simulink model "vmr_rwd_fix_leftarm"  (R2015a)
settings: Solver=ode4  SolverMode=MultiTasking  StartTime=0.0  StopTime=inf  FixedStep=BKIN_STEP_TIME  RelTol=1e-3
StartFcn:
  |  warndlg('Dexterit-E models cannot run under simulation. Please compile your model and run it from within Dexterit-E.');set_param(bdroot,'SimulationCommand','stop')
model workspace (MAT data in the model file):
  BKIN_STEP_TIME = 0.00025
  col_x = 1
  col_y = 2
  E_TARGET_ON = 3
  LOGICAL_RADIUS = 4
  START_TARGET_COL = 1
  END_TARGET_COL = 2
  ROTATION_CENTER = 3
  MAXREACHTIME_COL = 5
  ROTATION_TYPE = 7
  ROTATION = 8
  DELAY_POSTTRIAL_COL = 6
  E_STAY_CENTER = 2
  VISUAL_RADIUS = 3
  COLOR = 5
  K_SCORETEXT_ROW = 1
  LABEL_HEIGHT = 8
  HITCOLOR = 6
  E_HIT_TARGET = 5
  E_MISS_TARGET = 9
  K_REWARD_VAL = 2
  K_TONE_HIT_DURATION = 4
  K_TONE_HIT_FREQUENCY = 5
  K_VIS_RAD = 6
  E_REWARD = 6
  WAIT_AT_START_COL = 4
  LABEL = 7
  K_RETURN_RING_ROW = 7
  STROKE_WIDTH = 9
  STROKE_COLOR = 10
  K_SCORE_TIME = 8
  HAND_VIS_COL = 9
  CLAMP_COL = 10
  DO_REWARD_COL = 11
  K_TONE_NEUTRAL_DURATION = 10
  K_TONE_NEUTRAL_FREQUENCY = 11
  E_NEUTRAL_FDBK = 10
  E_SHOW_SCORE = 17
  DISPLAY_TRIAL_COL = 12
  K_INSTRUCT_TIME = 9
  E_SHOW_INSTRUCT = 18
  INSTRUCT_PAUSE_BTN = 2
  K_LEFTHAND_TGT = 12
  K_ROBOT_RAMP_TIME = 14
  K_ROBOT_MOVE_TIME = 15
  K_FIX_LEFTHAND = 13
  BKIN_KINEMATIC_FRAME_SIZE = 400
  E_NO_EVENT = 0
  K_UNUSED = 3
  ROTATED_COLOR = 11
undefined symbols (not defined in the file or in its folder): slselsubs
libraries: Video x9, slrtlib x7, General x3, KINARM_general x2, KINARM_loads x2, simulink x1, xpcnilib x1
(part 1 of 2)
CloseFcn:
  | rtwprivate ssgencode ModelCloseRequest b2lab2d
settings Model: ModifiedComment=chris -- Wed Feb 16 09:18:30 2005 -- Version 1.1384  ModifiedHistory=Feb 16/05 - Add error repeat, add offset ramp  ExtModeArmWhenConnect=off  ExtModeLogAll=off  Creator=Chris Grebeldinger  LastModifiedBy=User
settings SolverCC: EnableConcurrentExecution=on  AutoInsertRateTranBlk=on
settings DataIOCC: LimitDataPoints=off  SignalLoggingSaveFormat=ModelDataLogs  SaveOutput=off  SaveTime=off  SignalLoggingName=sigsOut
settings OptimizationCC: BlockReduction=off  BooleanDataType=off  OptimizeBlockIOStorage=off  BufferReuse=off  GlobalBufferReuse=off  ExpressionFolding=off  ExpressionDepthLimit=2147483647  LocalBlockOutputs=off  InitFltsAndDblsToZero=on
settings DebuggingCC: SaveWithParameterizedLinksMsg=none  UnderspecifiedInitializationDetection=Classic  MergeDetectMultiDrivingBlocksExec=none  SignalResolutionControl=TryResolveAllWithWarning  MultiTaskDSMMsg=warning  FcnCallInpInsideContextMsg=UseLocalSettings  StateNameClashWarn=warning  StrictBusMsg=ErrorOnBusTreatedAsVector
settings HardwareCC: ProdIntDivRoundTo=Zero  ProdEndianess=LittleEndian  ProdLongLongMode=on  ProdHWDeviceType=Generic->32-bit x86 compatible  TargetHWDeviceType=32-bit Generic
settings SFSimCC: SimParseCustomCode=off
settings RTWCC: SystemTargetFile=slrt.tlc  TemplateMakefile=slrt_default_tmf  Description=Simulink Real-Time  CustomSourceCode="#include \"stdio.h\""  RTWCompilerOptimization=on
settings CodeAppCC: MaxIdLength=63
settings SimulinkRealTimeCC: TargetFcnLib=ansi_tfl_tmw.mat  GeneratePreprocessorConditionals=Disable all  xPCisDownloadable=off

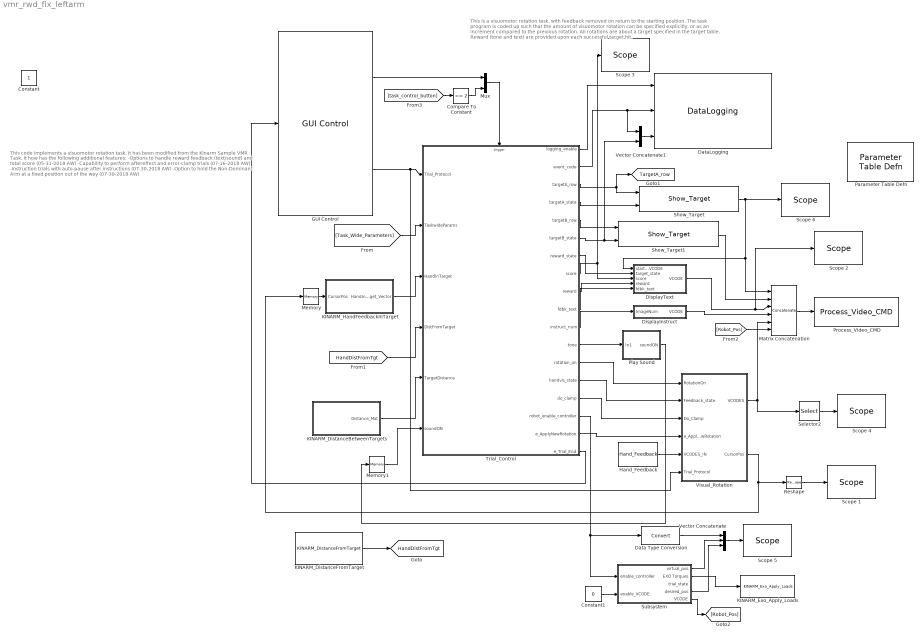
== system vmr_rwd_fix_leftarm ==
  note: This code implements a visuomotor rotation task. It has been modified from the Kinarm Sample VMR Task. It how has the following additional features:
      |
      | -Options to handle reward feedback (text/sound) and total score (05-31-2018 AW)
      | -Capability to perform aftereffect and error-clamp trials (07-16-2018 AW)
      | -Instruction trials with auto-pause after instructions (07-30-2018 AW)
      | -Option to hold the Non-Dominant Arm at a fixed position out of the way (07-30-2018 AW)
  note: This is a visuomotor rotation task, with feedback removed on return to the starting position.
      | The task program is coded up such that the amount of visuomotor rotation can be specified explicitly, or as an increment compared to the previous rotation.
      | All rotations are about a target specified in the target table.
      |
      | Reward (tone and text) are provided upon each successful target hit.
  Compare To Constant : simulink/Logic and Bit Operations/Compare To Constant  relop===  const=2  OutDataTypeStr=boolean
  Constant1 : Constant  Value=0  OutDataTypeStr=boolean
  Data Type Conversion : DataTypeConversion
  DataLogging : General/DataLogging  log_event_codes=on  log_analog_inputs=on  show_time_remaining=off
  DisplayInstruct : Subsystem
  DisplayText : Subsystem
  GUI Control : General/GUI Control  target_type_str=Circle  Target_Type=1  XYcols=[1 2]  Vcols=3  Lcols=4  indices_padding=[0 0 0 0;0 0 0 0]  task_version=1.0  show_repeat_trial_flag=off  target_table_rows=32  load_table_rows=20  tp_table_rows=100
  Hand_Feedback : KINARM_general/Hand_Feedback  feedback_cntl_src=none
  KINARM_DistanceBetweenTargets : Subsystem
  KINARM_DistanceFromTarget : KINARM_general/KINARM_DistanceFromTarget  use_dominant_hand=on
  KINARM_Exo_Apply_Loads : KINARM_loads/KINARM_Exo_Apply_Loads  up_duration=1500  down_duration=1500  max_torque=8  limit_motors=off
  KINARM_HandFeedbackInTarget : Subsystem  AncestorBlock=KINARM_general/KINARM_HandInTarget  mask(KINARM_HandInTarget){use_dominant_hand=on, target_type=Circle, num_states=1, attribcol1=4, attribcol2=3, attribcol3=3, attribcol4=3}
      mask prompts: use_dominant_hand "Dominant Hand?"; target_type "Type of Target"; num_states "Number of Target States"; attribcol1 "State 1 Target Table Column(s)"; attribcol2 "State 2 Target Table Column(s)"; attribcol3 "State 3 Target Table Column(s)"; attribcol4 "State 4 Target Table Column(s)"
      mask help: This block returns a vector or array corresponding to the Target_Table rows indicating whether the specified hand is in (=1) or out (=0) of each of the targets.
      mask init:
      | num_states=str2num(get_param(gcb, 'num_states'));
      | columntext='(columns: ';
      | 
      | for i=1:num_states
      | 	varname=['attribcol' num2str(i)];
      | 	if i>1
      | 		columntext=[columntext, '; '];
      | 	end
      | 	columntext=[columntext, get_param(gcb, varname)];
      | end
      | columntext=strvcat([columntext ')'],' ', ' ');
      | 
      | output_block=char(find_system(gcb,'LookUnderMasks','all','FollowLinks','on','SearchDepth',1,'BlockType','Outport'));
      | outputname=get_param(output_block,'Name');
      | 
      | % Select only the desired states for output. The output port is also renamed to reflect 
      | % whether the output is a vector (in the case of a single state) or an array (of vectors, 
      | % one for each of multiple states).
      | if num_states == 1
      | 	set_param([gcb '/Selected States'], 'Value', '[1]');
      | 	set_param(output_block, 'Name', 'HandInTarget_Vector');
      | elseif num_states == 2
      | 	set_param([gcb '/Selected States'], 'Value', '[1,2]');
      | 	set_param(output_block, 'Name', 'HandInTarget_Array');
      | elseif num_states == 3
      | 	set_param([gcb '/Selected States'], 'Value', '[1,2,3]');
      | 	set_param(output_block, 'Name', 'HandInTarget_Array');
      | else
      | 	set_param([gcb '/Selected States'], 'Value', '[1,2,3,4]');
      | 	set_param(output_block, 'Name', 'HandInTarget_Array');
      | end
      mask Help:
      | Used to determine if the hand (finger-tip) is in any of the targets in the Target_Table.
      | <P>
      | <B><I>Use of this block requires that the DataLogging block (General library) be set to log KINARM data.</I></B>
      | 
      | <H2>Library </H2>
      | KINARM_general (sub-library)
      | 
      | <H2>Description </H2>
      | This block returns a vector or array corresponding to the Target_Table rows indicating whether the specified hand (i.e. finger-tip) is in or out of each of the targets.  Each element in the output vector or output array will be either a 0 (hand not in target) or a 1 (hand in target).
      | <P>
      | A vector is returned if only one target state is specified in each target row (see Parameters and Dialog Box), with each index of the vector corresponding to a row in the target table.  An array is returned if more than one target state is specified in a target row, with each row of the array corresponding to a target row and each column corresponding to the nth target state specified in each target row.
      | <P>
      | The output vector or array is typically used by a stateflow chart to affect behavior of the system.  Because this block returns hand-in-target information for all targets in the target table, multiple targets can be monitored at once (i.e. the stateflow chart could have certain transitions that occur if the hand is in one target and other transitions if it is in a different target).  Likewise, because this block returns hand-in-target information for multiple states of a single target, those multiple states can be monitored simultaneously.
      | <P>
      | Because the KINARM_HandInTarget block returns information for only one hand, two copies of this block are required if information for both hands is desired.
      | <P>
      | 
      | <H2>Parameters and Dialog Box</H2>
      | <B>Dominant Hand?:</B> this box determines which hand is used by this block : dominant hand position (checked box) or the non-dominant hand position (unchecked box).  (Note: if the end-user wants to know about both the dominant hand and the non-dominant hand, then 2 separate copies of this block are requried, one for each hand.)
      | <P>
      | <B>Type of Target:</B> Enter the type of target specified in the target table:
      | <P>
      | <B>Number of Target States:</B> Enter the number of target states specified in each target row.  Up to four target states are allowed per target row.
      | <P>
      | <B>State <n> Target Table Columns:</B> Enter the columns in the Target Table that specify the relevant target attributes.  Do this for each target state.
      | For a circle, enter the columns corresponding to logical radius (e.g. 4)
      | <BR>For an ellipse, enter the columns corresponding to major radius, minor radius, rotation angle (e.g. [4, 5, 6]).
      | <BR>For a rectangle, enter the columns corresponding to length, height, and rotation angle (e.g. [4, 5, 6]).
      | <BR>For a line, enter the columns corresponding to stroke width, endpoint in x, and endpoint in y (e.g. [3, 4, 5]).
      | <BR>For a triangle, enter the columns corresponding to length, height, peak offset, and rotation angle (e.g. [4, 5, 6, 7]).
      | 
      | <H2>Examples</H2>
      | <B>Example 1.</B>  Suppose a target row will be used to define 1 state for a circle type target and the radius of the visual target is the same radius to be used for determination of hand-in-target.  The related Target Table column is: column 6 = radius.  For this example, "State 1 Target Table Columns" would equal [6].
      | <P>
      | 
      | <B>Example 2.</B>  Suppose a target row will be used to define 1 state for a circle type target, but the radius of the visual target will be different than the radius to be used for determination of hand-in-target.  This option allows independent control over the size of the visual target versus the accuracy needed to be considered "in the target".  The related Target Table columns are: column 6 = radius1 (i.e. radius to target to be drawn); column 7 = radius2 (i.e. radius to be used for hand-in-target) .  For this example, "State 1 Target Table Columns" would equal [7].
      | <P>
      | <B>Example 3.</B>  Suppose a target row will be used to define 2 states for a circle type target, where the radius of the visual target will be a constant, but depending on the state of the system, one of 2 other and different radii will be used for determination of hand-in-target.  The related Target Table columns are: column 6 = radius1 (i.e. radius to target to be drawn); column 7 = radius2 (i.e. radius to be used for hand-in-target for state 1); column 8 = radius3 (i.e. radius to be used for hand-in-target for state 2).  For this example, "State 1 Target Table Columns" would equal [7], while "State 2 Target Table Columns" would equal [8].
      | <P>
      | 
      | <H2>Related Blocks </H2>
      | DataLogging
      mask TypeOptions target_type: Circle | Ellipse | Rectangle | Line | Triangle
      mask Callback target_type:
      | target_type=get_param(gcb, 'target_type');
      | attribcol1=[str2num(get_param(gcb, 'attribcol1')) 0 0 0 0 0 0];
      | attribcol2=[str2num(get_param(gcb, 'attribcol2')) 0 0 0 0 0 0];
      | attribcol3=[str2num(get_param(gcb, 'attribcol3')) 0 0 0 0 0 0];
      | attribcol4=[str2num(get_param(gcb, 'attribcol4')) 0 0 0 0 0 0];
      | switch target_type(1:3)
      | 	case 'Cir'
      | 		numcol=1;
      | 	case 'Ell'
      | 		numcol=3;
      |     case 'Rec'
      |         numcol=3;
      |     case 'Lin'
      |         numcol=3;
      |     case 'Tri'
      |         numcol=4;
      | 	otherwise
      | 		numcol=1;
      | end
      | if numcol==1
      | 	set_param(gcb, 'attribcol1', num2str(attribcol1(1)));
      | 	set_param(gcb, 'attribcol2', num2str(attribcol2(1)));
      | 	set_param(gcb, 'attribcol3', num2str(attribcol3(1)));
      | 	set_param(gcb, 'attribcol4', num2str(attribcol4(1)));
      | else
      | 	set_param(gcb, 'attribcol1', ['[' num2str(attribcol1(1:numcol)) ']']);
      | 	set_param(gcb, 'attribcol2', ['[' num2str(attribcol2(1:numcol)) ']']);
      | 	set_param(gcb, 'attribcol3', ['[' num2str(attribcol3(1:numcol)) ']']);
      | 	set_param(gcb, 'attribcol4', ['[' num2str(attribcol4(1:numcol)) ']']);
      | end
      mask TypeOptions num_states: 1 | 2 | 3 | 4
      mask Callback num_states:
      | num_states = str2num(get_param(gcb, 'num_states'));
      | vis = get_param(gcb, 'MaskVisibilities');
      | 
      | % Select only the desired states for output. The output port is also renamed to reflect
      | % whether the output is a vector (in the case of a single state) or an array (of vectors,
      | % one for each of multiple states).
      | output_block=char(find_system(gcb, 'LookUnderMasks', 'all', 'FollowLinks', 'on', 'SearchDepth', 1, 'BlockType', 'Outport'));
      | 
      | if num_states == 1
      | 	set_param([gcb '/Selected States'], 'Value', '[1]');
      | 	set_param(output_block, 'Name', 'HandInTarget_Vector');
      | 	vis{5} = 'off';
      | 	vis{6} = 'off';
      | 	vis{7} = 'off';
      | elseif num_states == 2
      | 	set_param([gcb '/Selected States'], 'Value', '[1,2]');
      | 	set_param(output_block, 'Name', 'HandInTarget_Array');
      | 	vis{5} = 'on';
      | 	vis{6} = 'off';
      | 	vis{7} = 'off';
      | elseif num_states == 3
      | 	set_param([gcb '/Selected States'], 'Value', '[1,2,3]');
      | 	set_param(output_block, 'Name','HandInTarget_Array');
      | 	vis{5} = 'on';
      | 	vis{6} = 'on';
      | 	vis{7} = 'off';
      | else
      | 	set_param([gcb '/Selected States'], 'Value', '[1,2,3,4]');
      | 	set_param(output_block, 'Name', 'HandInTarget_Array');
      | 	vis{5} = 'on';
      | 	vis{6} = 'on';
      | 	vis{7} = 'on';
      | end
      | set_param(gcb, 'MaskVisibilities', vis);
      | 
      | target_type=get_param(gcb, 'target_type');
      | attribcol1=[str2num(get_param(gcb, 'attribcol1')) 0 0 0 0 0 0];
      | attribcol2=[str2num(get_param(gcb, 'attribcol2')) 0 0 0 0 0 0];
      | attribcol3=[str2num(get_param(gcb, 'attribcol3')) 0 0 0 0 0 0];
      | attribcol4=[str2num(get_param(gcb, 'attribcol4')) 0 0 0 0 0 0];
      | switch target_type(1:3)
      | 	case 'Cir'
      | 		numcol=1;
      | 	case 'Ell'
      | 		numcol=3;
      |     case 'Rec'
      |         numcol=3;
      |     case 'Lin'
      |         numcol=3;
      |     case 'Tri'
      |         numcol=4;
      | 	otherwise
      | 		numcol=1;
      | end
      | if numcol==1
      | 	set_param(gcb, 'attribcol1', num2str(attribcol1(1)));
      | 	set_param(gcb, 'attribcol2', num2str(attribcol2(1)));
      | 	set_param(gcb, 'attribcol3', num2str(attribcol3(1)));
      | 	set_param(gcb, 'attribcol4', num2str(attribcol4(1)));
      | else
      | 	set_param(gcb, 'attribcol1', ['[' num2str(attribcol1(1:numcol)) ']']);
      | 	set_param(gcb, 'attribcol2', ['[' num2str(attribcol2(1:numcol)) ']']);
      | 	set_param(gcb, 'attribcol3', ['[' num2str(attribcol3(1:numcol)) ']']);
      | 	set_param(gcb, 'attribcol4', ['[' num2str(attribcol4(1:numcol)) ']']);
      | end
      mask Callback attribcol1:
      | target_type=get_param(gcb, 'target_type');
      | attribcol1=[str2num(get_param(gcb, 'attribcol1')) 0 0 0 0 0 0];
      | attribcol2=[str2num(get_param(gcb, 'attribcol2')) 0 0 0 0 0 0];
      | attribcol3=[str2num(get_param(gcb, 'attribcol3')) 0 0 0 0 0 0];
      | attribcol4=[str2num(get_param(gcb, 'attribcol4')) 0 0 0 0 0 0];
      | switch target_type(1:3)
      | 	case 'Cir'
      | 		numcol=1;
      | 	case 'Ell'
      | 		numcol=3;
      |     case 'Rec'
      |         numcol=3;
      |     case 'Lin'
      |         numcol=3;
      |     case 'Tri'
      |         numcol=4;
      | 	otherwise
      | 		numcol=1;
      | end
      | if numcol==1
      | 	set_param(gcb, 'attribcol1', num2str(attribcol1(1)));
      | 	set_param(gcb, 'attribcol2', num2str(attribcol2(1)));
      | 	set_param(gcb, 'attribcol3', num2str(attribcol3(1)));
      | 	set_param(gcb, 'attribcol4', num2str(attribcol4(1)));
      | else
      | 	set_param(gcb, 'attribcol1', ['[' num2str(attribcol1(1:numcol)) ']']);
      | 	set_param(gcb, 'attribcol2', ['[' num2str(attribcol2(1:numcol)) ']']);
      | 	set_param(gcb, 'attribcol3', ['[' num2str(attribcol3(1:numcol)) ']']);
      | 	set_param(gcb, 'attribcol4', ['[' num2str(attribcol4(1:numcol)) ']']);
      | end
      mask Callback attribcol2:
      | target_type=get_param(gcb, 'target_type');
      | attribcol1=[str2num(get_param(gcb, 'attribcol1')) 0 0 0 0 0 0];
      | attribcol2=[str2num(get_param(gcb, 'attribcol2')) 0 0 0 0 0 0];
      | attribcol3=[str2num(get_param(gcb, 'attribcol3')) 0 0 0 0 0 0];
      | attribcol4=[str2num(get_param(gcb, 'attribcol4')) 0 0 0 0 0 0];
      | switch target_type(1:3)
      | 	case 'Cir'
      | 		numcol=1;
      | 	case 'Ell'
      | 		numcol=3;
      |     case 'Rec'
      |         numcol=3;
      |     case 'Lin'
      |         numcol=3;
      |     case 'Tri'
      |         numcol=4;
      | 	otherwise
      | 		numcol=1;
      | end
      | if numcol==1
      | 	set_param(gcb, 'attribcol1', num2str(attribcol1(1)));
      | 	set_param(gcb, 'attribcol2', num2str(attribcol2(1)));
      | 	set_param(gcb, 'attribcol3', num2str(attribcol3(1)));
      | 	set_param(gcb, 'attribcol4', num2str(attribcol4(1)));
      | else
      | 	set_param(gcb, 'attribcol1', ['[' num2str(attribcol1(1:numcol)) ']']);
      | 	set_param(gcb, 'attribcol2', ['[' num2str(attribcol2(1:numcol)) ']']);
      | 	set_param(gcb, 'attribcol3', ['[' num2str(attribcol3(1:numcol)) ']']);
      | 	set_param(gcb, 'attribcol4', ['[' num2str(attribcol4(1:numcol)) ']']);
      | end
      mask Callback attribcol3:
      | target_type=get_param(gcb, 'target_type');
      | attribcol1=[str2num(get_param(gcb, 'attribcol1')) 0 0 0 0 0 0];
      | attribcol2=[str2num(get_param(gcb, 'attribcol2')) 0 0 0 0 0 0];
      | attribcol3=[str2num(get_param(gcb, 'attribcol3')) 0 0 0 0 0 0];
      | attribcol4=[str2num(get_param(gcb, 'attribcol4')) 0 0 0 0 0 0];
      | switch target_type(1:3)
      | 	case 'Cir'
      | 		numcol=1;
      | 	case 'Ell'
      | 		numcol=3;
      |     case 'Rec'
      |         numcol=3;
      |     case 'Lin'
      |         numcol=3;
      |     case 'Tri'
      |         numcol=4;
      | 	otherwise
      | 		numcol=1;
      | end
      | if numcol==1
      | 	set_param(gcb, 'attribcol1', num2str(attribcol1(1)));
      | 	set_param(gcb, 'attribcol2', num2str(attribcol2(1)));
      | 	set_param(gcb, 'attribcol3', num2str(attribcol3(1)));
      | 	set_param(gcb, 'attribcol4', num2str(attribcol4(1)));
      | else
      | 	set_param(gcb, 'attribcol1', ['[' num2str(attribcol1(1:numcol)) ']']);
      | 	set_param(gcb, 'attribcol2', ['[' num2str(attribcol2(1:numcol)) ']']);
      | 	set_param(gcb, 'attribcol3', ['[' num2str(attribcol3(1:numcol)) ']']);
      | 	set_param(gcb, 'attribcol4', ['[' num2str(attribcol4(1:numcol)) ']']);
      | end
      mask Callback attribcol4:
      | target_type=get_param(gcb, 'target_type');
      | attribcol1=[str2num(get_param(gcb, 'attribcol1')) 0 0 0 0 0 0];
      | attribcol2=[str2num(get_param(gcb, 'attribcol2')) 0 0 0 0 0 0];
      | attribcol3=[str2num(get_param(gcb, 'attribcol3')) 0 0 0 0 0 0];
      | attribcol4=[str2num(get_param(gcb, 'attribcol4')) 0 0 0 0 0 0];
      | switch target_type(1:3)
      | 	case 'Cir'
      | 		numcol=1;
      | 	case 'Ell'
      | 		numcol=3;
      |     case 'Rec'
      |         numcol=3;
      |     case 'Lin'
      |         numcol=3;
      |     case 'Tri'
      |         numcol=4;
      | 	otherwise
      | 		numcol=1;
      | end
      | if numcol==1
      | 	set_param(gcb, 'attribcol1', num2str(attribcol1(1)));
      | 	set_param(gcb, 'attribcol2', num2str(attribcol2(1)));
      | 	set_param(gcb, 'attribcol3', num2str(attribcol3(1)));
      | 	set_param(gcb, 'attribcol4', num2str(attribcol4(1)));
      | else
      | 	set_param(gcb, 'attribcol1', ['[' num2str(attribcol1(1:numcol)) ']']);
      | 	set_param(gcb, 'attribcol2', ['[' num2str(attribcol2(1:numcol)) ']']);
      | 	set_param(gcb, 'attribcol3', ['[' num2str(attribcol3(1:numcol)) ']']);
      | 	set_param(gcb, 'attribcol4', ['[' num2str(attribcol4(1:numcol)) ']']);
      | end
      mask Display:
      | disp(columntext)
      | port_label('output',1,outputname)
  Matrix Concatenation : Concatenate  NumInputs=6  Mode=Multidimensional array
  Memory : Memory  InheritSampleTime=on
  Memory1 : Memory  LinearizeMemory=on
  Mux : Mux  Inputs=2
  Parameter Table Defn : General/Parameter Table Defn  ShowInLibBrowser=0
  Play Sound : Subsystem
  Process_Video_CMD : Video/Process_Video_CMD  video_delay=50
  Reshape : Reshape
  Scope 1 : slrtlib/Displays and Logging/Scope   scopeno=6  scopetype=Target  autostart=on  viewmode=Numerical  formatstr='%15.6f'  grid=on  ylimits=[0,0]  nosamples=250  noprepostsamples=0  interleave=1  triggermode=FreeRun  triggersignal=1  trigsignalfromport=off  triggerlevel=0.0  triggerslope=Either  triggerscope=1  triggersample=0  filename=data.dat  mode=Lazy  writesize=512  autorestart=off  dynamicfilemode=off  maxwritefilesize=512*1024^2
  Scope 2 : slrtlib/Displays and Logging/Scope   scopeno=1  scopetype=Target  autostart=on  viewmode=Numerical  formatstr='%15.6f'  grid=on  ylimits=[0,0]  nosamples=250  noprepostsamples=0  interleave=1  triggermode=FreeRun  triggersignal=1  trigsignalfromport=off  triggerlevel=0.0  triggerslope=Either  triggerscope=1  triggersample=0  filename=data.dat  mode=Lazy  writesize=512  autorestart=off  dynamicfilemode=off  maxwritefilesize=512*1024^2
  Scope 3 : slrtlib/Displays and Logging/Scope   scopeno=3  scopetype=Target  autostart=on  viewmode=Numerical  formatstr='%15.6f'  grid=on  ylimits=[0,0]  nosamples=250  noprepostsamples=0  interleave=1  triggermode=FreeRun  triggersignal=1  trigsignalfromport=off  triggerlevel=0.0  triggerslope=Either  triggerscope=1  triggersample=0  filename=data.dat  mode=Lazy  writesize=512  autorestart=off  dynamicfilemode=off  maxwritefilesize=512*1024^2
  Scope 4 : slrtlib/Displays and Logging/Scope   scopeno=5  scopetype=Target  autostart=on  viewmode=Numerical  formatstr='%15.6f'  grid=on  ylimits=[0,0]  nosamples=250  noprepostsamples=0  interleave=1  triggermode=FreeRun  triggersignal=1  trigsignalfromport=off  triggerlevel=0.0  triggerslope=Either  triggerscope=1  triggersample=0  filename=data.dat  mode=Lazy  writesize=512  autorestart=off  dynamicfilemode=off  maxwritefilesize=512*1024^2
  Scope 5 : slrtlib/Displays and Logging/Scope   scopeno=2  scopetype=Target  autostart=on  viewmode=Numerical  formatstr='%15.6f'  grid=on  ylimits=[0,0]  nosamples=250  noprepostsamples=0  interleave=1  triggermode=FreeRun  triggersignal=1  trigsignalfromport=off  triggerlevel=0.0  triggerslope=Either  triggerscope=1  triggersample=0  filename=data.dat  mode=Lazy  writesize=512  autorestart=off  dynamicfilemode=off  maxwritefilesize=512*1024^2
  Scope 6 : slrtlib/Displays and Logging/Scope   scopeno=4  scopetype=Target  autostart=on  viewmode=Numerical  formatstr='%15.6f'  grid=on  ylimits=[0,0]  nosamples=250  noprepostsamples=0  interleave=1  triggermode=FreeRun  triggersignal=1  trigsignalfromport=off  triggerlevel=0.0  triggerslope=Either  triggerscope=1  triggersample=0  filename=data.dat  mode=Lazy  writesize=512  autorestart=off  dynamicfilemode=off  maxwritefilesize=512*1024^2
  Selector2 : Selector  NumberOfDimensions=2  InputPortWidth=70  IndexOptions=Index vector (dialog),Select all  Indices=1,1  OutputSizes=1,1
  Show_Target : Video/Show_Target  target_type=Circle  num_states=2  attribcol1=[COLOR 0 0 VISUAL_RADIUS]  attribcol2=[HITCOLOR 0 0 VISUAL_RADIUS]  attribcol3=[0 0 0 0]  attribcol4=[0 0 0 0]  attribcol5=[0 0 24 0]  stateindices_padding=[0 0 0 0 0 0 0;0 0 0 0 0 0 0;0 0 0 0 0 0 0;0 0 0 0 0 0 0;0 0 0 0 0 0 0]  source=dialog  opacity=100  target_display=Both subject and operator displays  num_col=4
  Show_Target1 : Video/Show_Target  target_type=Circle  num_states=3  attribcol1=[COLOR 0 0 VISUAL_RADIUS]  attribcol2=[HITCOLOR 0 0 VISUAL_RADIUS]  attribcol3=[ROTATED_COLOR 0 0 VISUAL_RADIUS]  attribcol4=[0 0 0 0]  attribcol5=[0 0 24 0]  stateindices_padding=[0 0 0 0 0 0 0;0 0 0 0 0 0 0;0 0 0 0 0 0 0;0 0 0 0 0 0 0;0 0 0 0 0 0 0]  source=dialog  opacity=100  target_display=Both subject and operator displays  num_col=4
  Subsystem : Subsystem
  Trial_Control : Stateflow chart  TreatAsAtomicUnit=on
  Vector Concatenate : Concatenate  NumInputs=3
  Vector Concatenate1 : Concatenate
  Visual_Rotation : Subsystem
  Constant : Constant  IOType=siggen
  tag scope: HandDistFromTgt=global, TargetA_row=global
  wires:
  Show_Target/1 -> Scope 6/1, Matrix Concatenation/1, DisplayText/1(start_tgt_VCODE)
  GUI Control/2 -> Visual_Rotation/6(Trial_Protocol), Trial_Control/1(Trial_Protocol)
  Trial_Control/18(e_Trial_End) -> GUI Control/1
  Trial_Control/4(targetA_state) -> Show_Target/2
  Trial_Control/3(targetA_row) -> Show_Target/1, [TargetA_row]
  Show_Target1/1 -> Matrix Concatenation/2
  Trial_Control/5(targetB_row) -> Show_Target1/1
  Trial_Control/6(targetB_state) -> Vector Concatenate1/2, Show_Target1/2
  Trial_Control/2(event_code) -> DataLogging/2, Vector Concatenate1/1
  Matrix Concatenation/1 -> Process_Video_CMD/1
  Hand_Feedback/1 -> Visual_Rotation/5(VCODES_IN)
  Visual_Rotation/2(CursorPos) -> Memory/1, Reshape/1
  KINARM_HandFeedbackInTarget/1(HandInTarget_Vector) -> Trial_Control/3(HandInTarget)
  Trial_Control/17(e_ApplyNewRotation) -> Visual_Rotation/4(e_ApplyNewRotation)
  Trial_Control/1(logging_enable) -> DataLogging/1
  Trial_Control/7(reward_state) -> DisplayText/2(target_state)
  Trial_Control/8(score) -> DisplayText/3(score), Scope 3/1
  [Task_Wide_Parameters] -> Trial_Control/2(TaskwideParams)
  [HandDistFromTgt] -> Trial_Control/4(DistFromTarget)
  KINARM_DistanceBetweenTargets/1(Distance_Mat) -> Trial_Control/5(TargetDistance)
  Trial_Control/9(reward) -> DisplayText/4(reward)
  Trial_Control/13(rotation_on) -> Visual_Rotation/1(RotationOn)
  Trial_Control/14(handvis_state) -> Visual_Rotation/2(Feedback_state)
  Reshape/1 -> Scope 1/1
  Memory/1 -> KINARM_HandFeedbackInTarget/1(CursorPos)
  Selector2/1 -> Scope 4/1
  KINARM_DistanceFromTarget/1 -> [HandDistFromTgt]
  Trial_Control/15(do_clamp) -> Visual_Rotation/3(Do_Clamp)
  DisplayInstruct/1(VCODE) -> Matrix Concatenation/4
  Trial_Control/11(instruct_num) -> DisplayInstruct/1(ImageNum)
  Trial_Control/10(fdbk_text) -> DisplayText/5(fdbk_text)
  Visual_Rotation/1(VCODES) -> Matrix Concatenation/5, Selector2/1
  DisplayText/1(VCODE) -> Scope 2/1, Matrix Concatenation/3
  GUI Control/1 -> Mux/1
  [task_control_button] -> Compare To Constant/1
  Compare To Constant/1 -> Mux/2
  Mux/1 -> Trial_Control/Trigger
  Subsystem/2(EXO Torques) -> KINARM_Exo_Apply_Loads/1
  Subsystem/1(virtual_pos) -> Vector Concatenate/2
  Trial_Control/16(robot_enable_controller) -> Data Type Conversion/1, Subsystem/1(enable_controller)
  Vector Concatenate/1 -> Scope 5/1
  Data Type Conversion/1 -> Vector Concatenate/1
  Subsystem/4(desired_pos) -> Vector Concatenate/3
  Constant1/1 -> Subsystem/2(enable_VCODE)
  Subsystem/5(VCODE) -> [Robot_Pos]
  [Robot_Pos] -> Matrix Concatenation/6
  Vector Concatenate1/1 -> DataLogging/3
  Trial_Control/12(tone) -> Play Sound/1(In1)
  Play Sound/1(soundON) -> Memory1/1
  Memory1/1 -> Trial_Control/6(soundON)

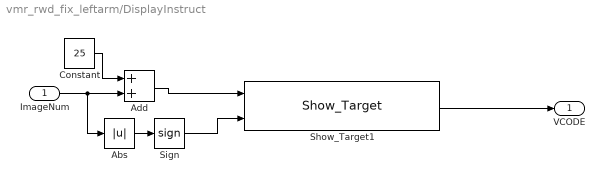
== system vmr_rwd_fix_leftarm/DisplayInstruct ==
  ImageNum : Inport
  Abs : Abs
  Add : Sum
  Constant : Constant  Value=25
  Show_Target1 : Video/Show_Target  target_type=Rectangle  num_states=1  attribcol1=[COLOR 0 0 VISUAL_RADIUS LABEL_HEIGHT 0]  attribcol2=[HITCOLOR 0 0 VISUAL_RADIUS 0 0]  attribcol3=[0 0 0 0 0 0]  attribcol4=[0 0 0 0 0 0]  attribcol5=[0 0 24 0 0 0]  stateindices_padding=[0 0 0 0 0;0 0 0 0 0;0 0 0 0 0;0 0 0 0 0;0 0 0 0 0]  source=dialog  opacity=100  target_display=Both subject and operator displays  num_col=6
  Sign : Signum
  VCODE : Outport
  wires:
  ImageNum/1 -> Add/2, Abs/1
  Abs/1 -> Sign/1
  Sign/1 -> Show_Target1/2
  Show_Target1/1 -> VCODE/1
  Add/1 -> Show_Target1/1
  Constant/1 -> Add/1

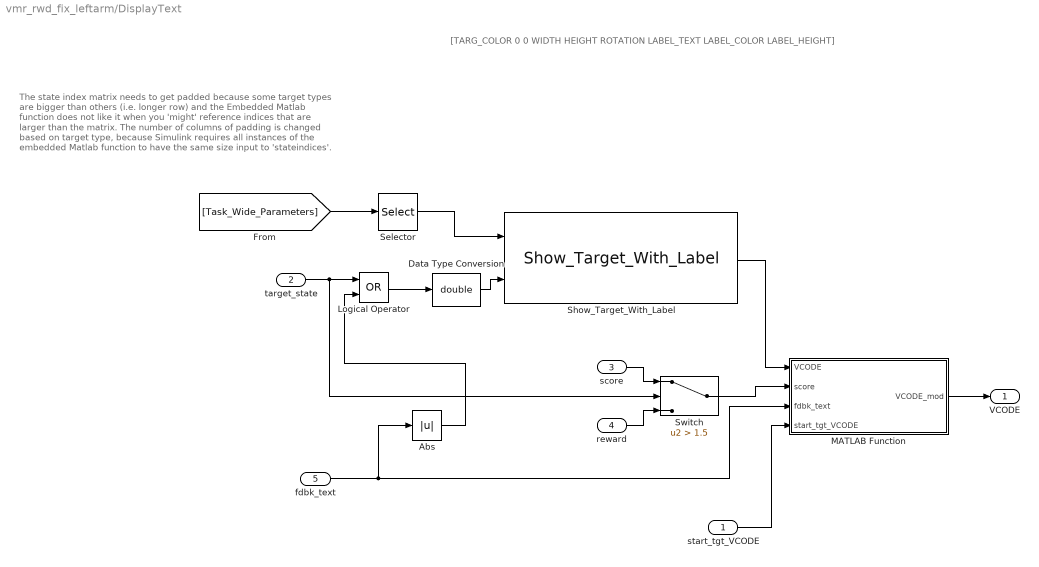
== system vmr_rwd_fix_leftarm/DisplayText ==
  note: [TARG_COLOR 0 0 WIDTH HEIGHT ROTATION LABEL_TEXT LABEL_COLOR LABEL_HEIGHT]
  note: The state index matrix needs to get padded because
      | some target types are bigger than others (i.e. longer row)
      | and the Embedded Matlab function does not like it when you
      |  'might' reference indices that are larger than the matrix.
      |
      | The number of columns of padding is changed based on target
      | type, because Simulink requires all instances of the embedded
      | Matlab function to have the same size input to 'stateindices'.
  start_tgt_VCODE : Inport  OutDataTypeStr=double
  target_state : Inport  Port=2  OutDataTypeStr=double
  score : Inport  Port=3  OutDataTypeStr=int32
  reward : Inport  Port=4  OutDataTypeStr=int32
  fdbk_text : Inport  Port=5  OutDataTypeStr=int32
  Abs : Abs
  Data Type Conversion : DataTypeConversion  OutDataTypeStr=double
  Logical Operator : Logic  Operator=OR  AllPortsSameDT=off  OutDataTypeStr=boolean
  MATLAB Function : MATLAB Function  TreatAsAtomicUnit=on
  Selector : Selector  Indices=[K_SCORETEXT_ROW]
  Show_Target_With_Label : Video/Show_Target_With_Label  target_type=Rectangle  num_states=1  attribcol1=[COLOR 0 0 VISUAL_RADIUS VISUAL_RADIUS 0 LABEL COLOR LABEL_HEIGHT]  attribcol2=[COLOR 0 0 VISUAL_RADIUS VISUAL_RADIUS 0 LABEL COLOR LABEL_HEIGHT]  attribcol3=[0 0 0 0 0 0 0 0 0]  attribcol4=[0 0 0 0 0 0 0 0 0]  attribcol5=[0 0 24 0 0 0 0 0 0]  stateindices_padding=[0 0;0 0;0 0;0 0;0 0]  source=dialog  opacity=100  target_display=Both subject and operator displays
  Switch : Switch  Criteria=u2 > Threshold  Threshold=1.5
  VCODE : Outport
  wires:
  target_state/1 -> Logical Operator/1, Switch/2
  Show_Target_With_Label/1 -> MATLAB Function/1(VCODE)
  MATLAB Function/1(VCODE_mod) -> VCODE/1
  score/1 -> Switch/1
  reward/1 -> Switch/3
  Switch/1 -> MATLAB Function/2(score)
  [Task_Wide_Parameters] -> Selector/1
  Selector/1 -> Show_Target_With_Label/1
  fdbk_text/1 -> Abs/1, MATLAB Function/3(fdbk_text)
  Abs/1 -> Logical Operator/2
  Logical Operator/1 -> Data Type Conversion/1
  Data Type Conversion/1 -> Show_Target_With_Label/2
  start_tgt_VCODE/1 -> MATLAB Function/4(start_tgt_VCODE)

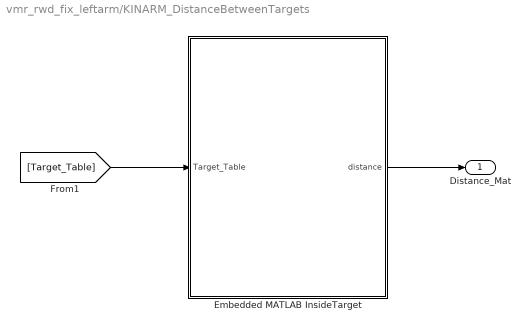
== system vmr_rwd_fix_leftarm/KINARM_DistanceBetweenTargets ==
  Embedded MATLAB InsideTarget : MATLAB Function  TreatAsAtomicUnit=on
  Distance_Mat : Outport
  wires:
  Embedded MATLAB InsideTarget/1(distance) -> Distance_Mat/1
  [Target_Table] -> Embedded MATLAB InsideTarget/1(Target_Table)

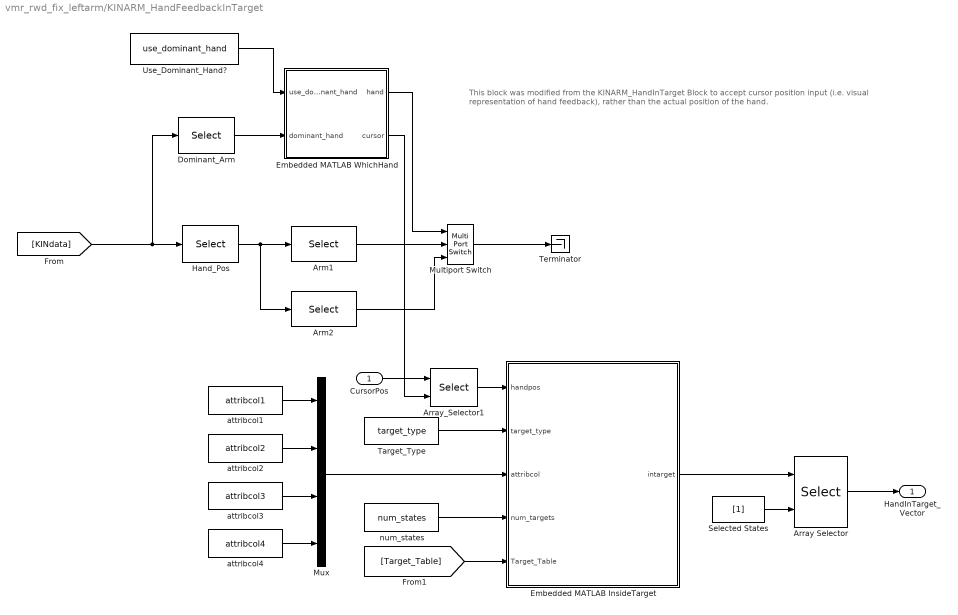
== system vmr_rwd_fix_leftarm/KINARM_HandFeedbackInTarget ==
  note: This block was modified from the KINARM_HandInTarget Block to accept cursor position input (i.e. visual
      | representation of hand feedback), rather than the actual position of the hand.
  CursorPos : Inport
  Arm1 : Selector  NumberOfDimensions=2  InputPortWidth=3  IndexOptions=Index vector (dialog),Select all  Indices=1,-1  OutputSizes=slselsubs([(-2),(-2)],1),slselsubs([(-2),(-2)],2)
  Arm2 : Selector  NumberOfDimensions=2  InputPortWidth=3  IndexOptions=Index vector (dialog),Select all  Indices=2,-1  OutputSizes=slselsubs([(-2),(-2)],1),slselsubs([(-2),(-2)],2)
  Array Selector : Selector  NumberOfDimensions=2  InputPortWidth=3  IndexOptions=Select all,Index vector (port)  Indices=-1,1  OutputSizes=slselsubs([(-2),(-2)],1),slselsubs([(-2),(-2)],2)
  Array_Selector1 : Selector  NumberOfDimensions=2  InputPortWidth=3  IndexOptions=Index vector (port),Select all  Indices=-1,1
  Dominant_Arm : Selector  NumberOfDimensions=2  InputPortWidth=3  IndexOptions=Index vector (dialog),Index vector (dialog)  Indices=[3],[1]  OutputSizes=slselsubs([(-2),(-2)],1),slselsubs([(-2),(-2)],2)
  Embedded MATLAB InsideTarget : MATLAB Function  TreatAsAtomicUnit=on
  Embedded MATLAB WhichHand : MATLAB Function  TreatAsAtomicUnit=on
  Hand_Pos : Selector  NumberOfDimensions=2  InputPortWidth=3  IndexOptions=Select all,Index vector (dialog)  Indices=-1,[23,24]  OutputSizes=slselsubs([(-2),(-2)],1),slselsubs([(-2),(-2)],2)
  Multiport Switch : MultiPortSwitch  Inputs=2
  Mux : Mux
  Selected States : Constant  Value=[1]
  Target_Type : Constant  Value=target_type
  Terminator : Terminator
  Use_Dominant_Hand? : Constant  Value=use_dominant_hand
  attribcol1 : Constant  Value=attribcol1
  attribcol2 : Constant  Value=attribcol2
  attribcol3 : Constant  Value=attribcol3
  attribcol4 : Constant  Value=attribcol4
  num_states : Constant  Value=num_states
  HandInTarget_Vector : Outport
  wires:
  Selected States/1 -> Array Selector/2
  num_states/1 -> Embedded MATLAB InsideTarget/4(num_targets)
  Mux/1 -> Embedded MATLAB InsideTarget/3(attribcol)
  attribcol4/1 -> Mux/4
  attribcol3/1 -> Mux/3
  attribcol2/1 -> Mux/2
  attribcol1/1 -> Mux/1
  Use_Dominant_Hand?/1 -> Embedded MATLAB WhichHand/1(use_dominant_hand)
  Embedded MATLAB WhichHand/1(hand) -> Multiport Switch/1
  Target_Type/1 -> Embedded MATLAB InsideTarget/2(target_type)
  Array Selector/1 -> HandInTarget_Vector/1
  [Target_Table] -> Embedded MATLAB InsideTarget/5(Target_Table)
  Embedded MATLAB InsideTarget/1(intarget) -> Array Selector/1
  Multiport Switch/1 -> Terminator/1
  Arm2/1 -> Multiport Switch/3
  Arm1/1 -> Multiport Switch/2
  Dominant_Arm/1 -> Embedded MATLAB WhichHand/2(dominant_hand)
  Hand_Pos/1 -> Arm2/1, Arm1/1
  [KINdata] -> Dominant_Arm/1, Hand_Pos/1
  CursorPos/1 -> Array_Selector1/1
  Array_Selector1/1 -> Embedded MATLAB InsideTarget/1(handpos)
  Embedded MATLAB WhichHand/2(cursor) -> Array_Selector1/2

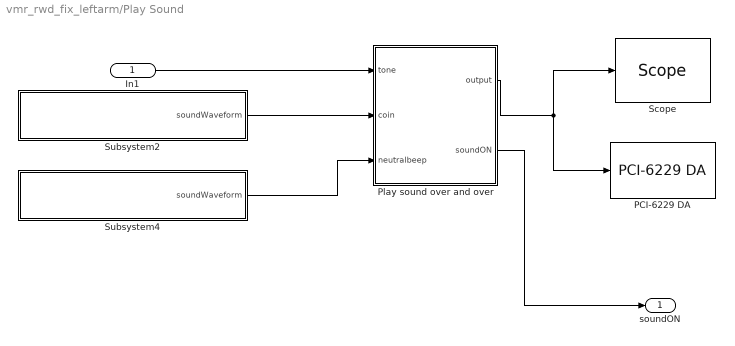
== system vmr_rwd_fix_leftarm/Play Sound ==
  In1 : Inport
  PCI-6229 DA : xpcnilib/D//A/M Series/PCI-6229 DA  channel=[1]  reset=[1]  initValue=[0]  sampletime=-1  slot=-1
  Play sound over and over : MATLAB Function  TreatAsAtomicUnit=on
  "Scope " : slrtlib/Displays and Logging/Scope   scopeno=7  scopetype=Target  autostart=on  viewmode=Graphical redraw  formatstr='%15.6f'  grid=on  ylimits=[0,0]  nosamples=4000  noprepostsamples=0  interleave=1  triggermode=FreeRun  triggersignal=1  trigsignalfromport=off  triggerlevel=0.0  triggerslope=Either  triggerscope=1  triggersample=0  filename=data.dat  mode=Lazy  writesize=512  autorestart=off  dynamicfilemode=off  maxwritefilesize=512*1024^2
  Subsystem2 : Subsystem  mask(Load Waveform Into Variable){fileName=coin}
      mask prompts: fileName "Name of .mat Data File (must be in current directory)"
      mask help: This block will load the .MAT file specified in the dialog, and put the first variable into a GoTo called 'soundWaveform'.
      mask init:
      | filenameFromMask = get_param(gcb, 'fileName');
      | 
      | try 
      | 	dataFromFile = load(filenameFromMask);
      | 	names = fieldnames(dataFromFile);
      | 	soundDataFromFile = dataFromFile.(names{1});
      | 	display(['Sound waveform from file ''' filenameFromMask ''' loaded.']);
      | catch ME
      | 	display(ME.message)
      | end
      mask Help:
      | Enter the name a .MAT file containing a single vector or matrix. The .MAT file must be located in the current directory.
      | 
      | The first variable from the .MAT file will be put into a Goto called 'soundWaveform'.
      mask Display: disp(['Load waveform from ''' filenameFromMask ''''])
  Subsystem4 : Subsystem  mask(Load Waveform Into Variable){fileName=neutralbeep}
      mask prompts: fileName "Name of .mat Data File (must be in current directory)"
      mask help: This block will load the .MAT file specified in the dialog, and put the first variable into a GoTo called 'soundWaveform'.
      mask init: same as vmr_rwd_fix_leftarm/Play Sound/Subsystem2
      mask Help:
      | Enter the name a .MAT file containing a single vector or matrix. The .MAT file must be located in the current directory.
      | 
      | The first variable from the .MAT file will be put into a Goto called 'soundWaveform'.
      mask Display: disp(['Load waveform from ''' filenameFromMask ''''])
  soundON : Outport
  wires:
  Play sound over and over/1(output) -> PCI-6229 DA/1, "Scope "/1
  Subsystem4/1(soundWaveform) -> Play sound over and over/3(neutralbeep)
  In1/1 -> Play sound over and over/1(tone)
  Subsystem2/1(soundWaveform) -> Play sound over and over/2(coin)
  Play sound over and over/2(soundON) -> soundON/1

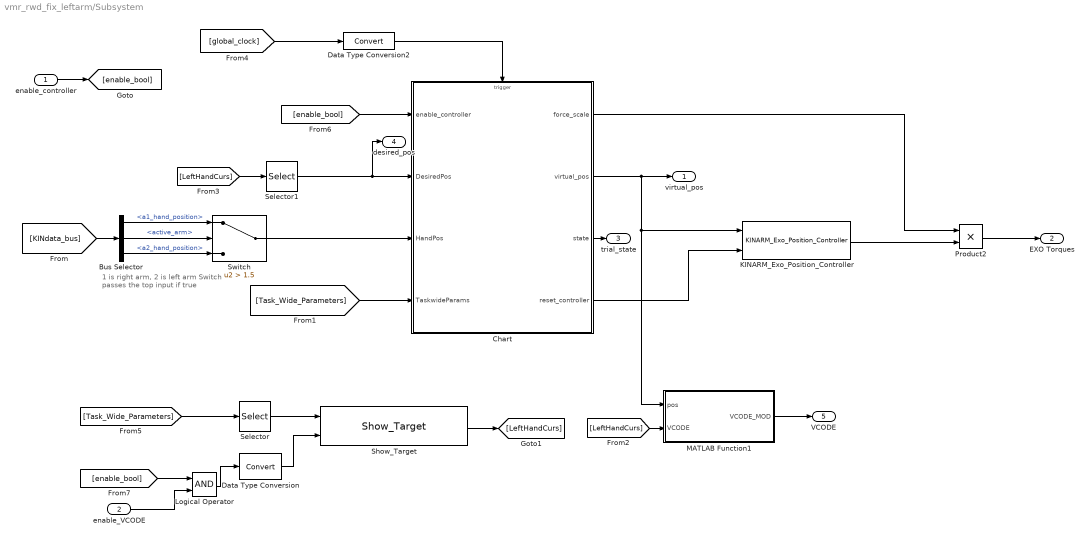
== system vmr_rwd_fix_leftarm/Subsystem ==
  note: 1 is right arm, 2 is left arm
      | Switch passes the top input if true
  enable_controller : Inport
  enable_VCODE : Inport  Port=2
  Bus Selector : BusSelector  OutputSignals=Robot1.a1_hand_position,KINDataGeneral.active_arm,Robot2.a2_hand_position
  Chart : Stateflow chart  TreatAsAtomicUnit=on
  Data Type Conversion : DataTypeConversion
  Data Type Conversion2 : DataTypeConversion
  KINARM_Exo_Position_Controller : KINARM_loads/KINARM_Exo_Position_Controller  use_dom_hand=off  KINARM_Type=Human  inertias_for_FF=KINARM robot & arm troughs & subject  angles_or_XY=End-point (global x/y)  sample_time=0.001
  Logical Operator : Logic  AllPortsSameDT=off  OutDataTypeStr=boolean
  MATLAB Function1 : MATLAB Function  TreatAsAtomicUnit=on
  Product2 : Product
  Selector : Selector  InputPortWidth=50  Indices=[12]
  Selector1 : Selector  InputPortWidth=70  Indices=[3 4]
  Show_Target : Video/Show_Target  target_type=Circle  num_states=1  attribcol1=[COLOR 0 0 VISUAL_RADIUS]  attribcol2=[6 6 0 3]  attribcol3=[0 0 0 0]  attribcol4=[0 0 0 0]  attribcol5=[0 0 24 0]  stateindices_padding=[0 0 0 0 0 0 0;0 0 0 0 0 0 0;0 0 0 0 0 0 0;0 0 0 0 0 0 0;0 0 0 0 0 0 0]  source=dialog  opacity=100  target_display=Both subject and operator displays  num_col=4
  Switch : Switch  Criteria=u2 > Threshold  Threshold=1.5
  virtual_pos : Outport
  EXO Torques : Outport  Port=2
  trial_state : Outport  Port=3
  desired_pos : Outport  Port=4
  VCODE : Outport  Port=5
  wires:
  [KINdata_bus] -> Bus Selector/1
  Bus Selector/2 -> Switch/2  "<active_arm>"
  [Task_Wide_Parameters] -> Chart/4(TaskwideParams)
  [global_clock] -> Data Type Conversion2/1
  Data Type Conversion2/1 -> Chart/Trigger
  Chart/2(virtual_pos) -> MATLAB Function1/1(pos), KINARM_Exo_Position_Controller/1, virtual_pos/1
  Switch/1 -> Chart/3(HandPos)
  Selector1/1 -> desired_pos/1, Chart/2(DesiredPos)
  KINARM_Exo_Position_Controller/1 -> Product2/2
  Product2/1 -> EXO Torques/1
  Chart/1(force_scale) -> Product2/1
  Chart/4(reset_controller) -> KINARM_Exo_Position_Controller/2
  Chart/3(state) -> trial_state/1
  enable_controller/1 -> [enable_bool]
  Bus Selector/1 -> Switch/1  "<a1_hand_position>"
  Bus Selector/3 -> Switch/3  "<a2_hand_position>"
  [Task_Wide_Parameters] -> Selector/1
  Selector/1 -> Show_Target/1
  [enable_bool] -> Chart/1(enable_controller)
  [enable_bool] -> Logical Operator/1
  Data Type Conversion/1 -> Show_Target/2
  Show_Target/1 -> [LeftHandCurs]
  MATLAB Function1/1(VCODE_MOD) -> VCODE/1
  enable_VCODE/1 -> Logical Operator/2
  Logical Operator/1 -> Data Type Conversion/1
  [LeftHandCurs] -> MATLAB Function1/2(VCODE)
  [LeftHandCurs] -> Selector1/1

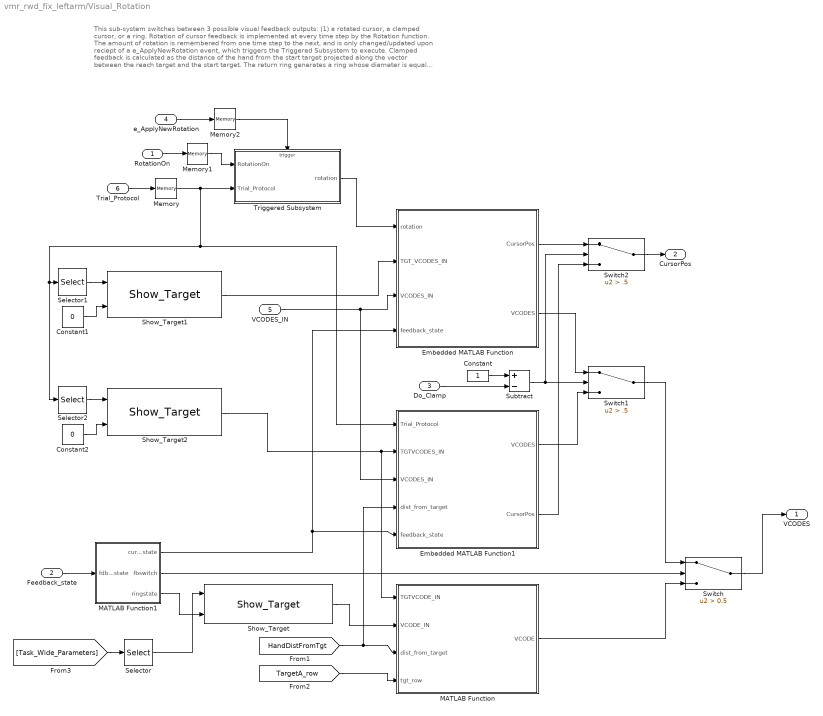
== system vmr_rwd_fix_leftarm/Visual_Rotation ==
  note: This sub-system switches between 3 possible visual feedback outputs: (1) a rotated cursor, a clamped cursor, or a ring.
      |
      | Rotation of cursor feedback is implemented at every time step by the Rotation function.
      | The amount of rotation is remembered from one time step to the next, and is only changed/updated
      | upon reciept of a e_ApplyNewRotation event, which triggers the Triggered Subsystem to execute.
      |
      | Clamped feedback is calculated as the distance of the hand from the start target projected along the vector between the
      | reach target and the start target.
      |
      | The return ring generates a ring whose diameter is equal to the distance of the hand from the start target.
      |
      | The memory blocks on the inputs to this block prevent a loop from occuring (i.e. if the output from here goes to
      | another block which then feeds back into this block, which forms a loop, which needs to be broken by the Memory block).
  RotationOn : Inport
  Feedback_state : Inport  Port=2
  Do_Clamp : Inport  Port=3
  e_ApplyNewRotation : Inport  Port=4
  VCODES_IN : Inport  Port=5
  Trial_Protocol : Inport  Port=6
  Constant : Constant
  Constant1 : Constant  Value=0
  Constant2 : Constant  Value=0
  Embedded MATLAB Function : MATLAB Function  TreatAsAtomicUnit=on
  Embedded MATLAB Function1 : MATLAB Function  TreatAsAtomicUnit=on
  MATLAB Function : MATLAB Function  TreatAsAtomicUnit=on
  MATLAB Function1 : MATLAB Function  TreatAsAtomicUnit=on
  Memory : Memory  InheritSampleTime=on
  Memory1 : Memory  InheritSampleTime=on
  Memory2 : Memory  InheritSampleTime=on
  Selector : Selector  Indices=[K_RETURN_RING_ROW]
  Selector1 : Selector  InputPortWidth=50  Indices=[ROTATION_CENTER]
  Selector2 : Selector  InputPortWidth=50  Indices=[START_TARGET_COL,END_TARGET_COL]
  Show_Target : Video/Show_Target  target_type=Circle  num_states=1  attribcol1=[COLOR STROKE_COLOR STROKE_WIDTH VISUAL_RADIUS]  attribcol2=[6 6 0 3]  attribcol3=[0 0 0 0]  attribcol4=[0 0 0 0]  attribcol5=[0 0 24 0]  stateindices_padding=[0 0 0 0 0 0 0;0 0 0 0 0 0 0;0 0 0 0 0 0 0;0 0 0 0 0 0 0;0 0 0 0 0 0 0]  source=dialog  opacity=100  target_display=Both subject and operator displays  num_col=4
  Show_Target1 : Video/Show_Target  target_type=Circle  num_states=1  attribcol1=[COLOR 0 0 VISUAL_RADIUS]  attribcol2=[6 6 0 3]  attribcol3=[0 0 0 0]  attribcol4=[0 0 0 0]  attribcol5=[0 0 24 0]  stateindices_padding=[0 0 0 0 0 0 0;0 0 0 0 0 0 0;0 0 0 0 0 0 0;0 0 0 0 0 0 0;0 0 0 0 0 0 0]  source=dialog  opacity=100  target_display=Both subject and operator displays  num_col=4
  Show_Target2 : Video/Show_Target  target_type=Circle  num_states=1  attribcol1=[COLOR 0 0 VISUAL_RADIUS]  attribcol2=[6 6 0 3]  attribcol3=[0 0 0 0]  attribcol4=[0 0 0 0]  attribcol5=[0 0 24 0]  stateindices_padding=[0 0 0 0 0 0 0;0 0 0 0 0 0 0;0 0 0 0 0 0 0;0 0 0 0 0 0 0;0 0 0 0 0 0 0]  source=dialog  opacity=100  target_display=Both subject and operator displays  num_col=4
  Subtract : Sum  Inputs=+-
  Switch : Switch  Criteria=u2 > Threshold  Threshold=0.5
  Switch1 : Switch  Criteria=u2 > Threshold  Threshold=.5
  Switch2 : Switch  Criteria=u2 > Threshold  Threshold=.5
  Triggered Subsystem : Subsystem  TreatAsAtomicUnit=on
  VCODES : Outport
  CursorPos : Outport  Port=2
  wires:
  Trial_Protocol/1 -> Memory/1
  VCODES_IN/1 -> Embedded MATLAB Function1/3(VCODES_IN), Embedded MATLAB Function/3(VCODES_IN)
  Memory/1 -> Triggered Subsystem/2(Trial_Protocol), Embedded MATLAB Function1/1(Trial_Protocol), Selector2/1, Selector1/1
  e_ApplyNewRotation/1 -> Memory2/1
  Triggered Subsystem/1(rotation) -> Embedded MATLAB Function/1(rotation)
  Memory2/1 -> Triggered Subsystem/Trigger
  RotationOn/1 -> Memory1/1
  Memory1/1 -> Triggered Subsystem/1(RotationOn)
  Switch/1 -> VCODES/1
  MATLAB Function/1(VCODE) -> Switch/3
  Feedback_state/1 -> MATLAB Function1/1(fdbkstate)
  [HandDistFromTgt] -> Embedded MATLAB Function1/4(dist_from_target), MATLAB Function/3(dist_from_target)
  [TargetA_row] -> MATLAB Function/4(tgt_row)
  Show_Target/1 -> MATLAB Function/2(VCODE_IN)
  [Task_Wide_Parameters] -> Selector/1
  Selector/1 -> Show_Target/1
  MATLAB Function1/3(ringstate) -> Show_Target/2
  Switch1/1 -> Switch/1
  Embedded MATLAB Function/2(VCODES) -> Switch1/1
  Embedded MATLAB Function1/1(VCODES) -> Switch1/3
  Embedded MATLAB Function/1(CursorPos) -> Switch2/1
  Switch2/1 -> CursorPos/1
  Embedded MATLAB Function1/2(CursorPos) -> Switch2/3
  MATLAB Function1/2(fbswitch) -> Switch/2
  MATLAB Function1/1(cursstate) -> Embedded MATLAB Function/4(feedback_state), Embedded MATLAB Function1/5(feedback_state)
  Subtract/1 -> Switch2/2, Switch1/2
  Do_Clamp/1 -> Subtract/2
  Constant/1 -> Subtract/1
  Selector1/1 -> Show_Target1/1
  Constant1/1 -> Show_Target1/2
  Show_Target1/1 -> Embedded MATLAB Function/2(TGT_VCODES_IN)
  Selector2/1 -> Show_Target2/1
  Constant2/1 -> Show_Target2/2
  Show_Target2/1 -> MATLAB Function/1(TGTVCODE_IN), Embedded MATLAB Function1/2(TGTVCODES_IN)

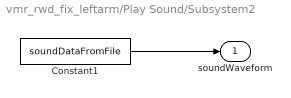
== system vmr_rwd_fix_leftarm/Play Sound/Subsystem2 ==
  Constant1 : Constant  Value=soundDataFromFile
  soundWaveform : Outport
  wires:
  Constant1/1 -> soundWaveform/1

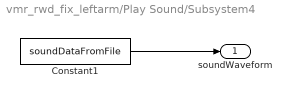
== system vmr_rwd_fix_leftarm/Play Sound/Subsystem4 ==
  Constant1 : Constant  Value=soundDataFromFile
  soundWaveform : Outport
  wires:
  Constant1/1 -> soundWaveform/1

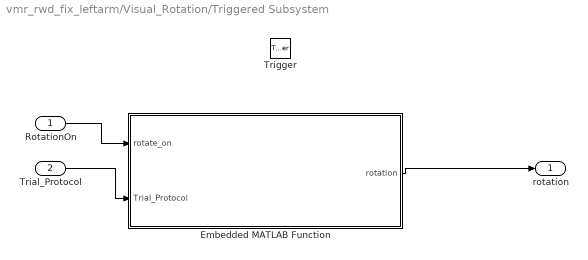
== system vmr_rwd_fix_leftarm/Visual_Rotation/Triggered Subsystem ==
  RotationOn : Inport
  Trial_Protocol : Inport  Port=2
  Trigger : TriggerPort  TriggerType=either
  Embedded MATLAB Function : MATLAB Function  TreatAsAtomicUnit=on
  rotation : Outport
  wires:
  Trial_Protocol/1 -> Embedded MATLAB Function/2(Trial_Protocol)
  Embedded MATLAB Function/1(rotation) -> rotation/1
  RotationOn/1 -> Embedded MATLAB Function/1(rotate_on)
